simulink model "sm_DynamicCompression"  (R2019b)
settings: Solver=FixedStepDiscrete  StartTime=0.0  StopTime=stop_time  RelTol=1e-3
InitFcn:
  | sm_callback_init
StopFcn:
  | sm_callback_stop
values from neighbouring files (symbols this model uses):
  a = 100*(r^2)    [InitializeCompressionSettings.m]    (also in sm_check_control_signals.m = registers(i).(supplied_fields{j}); sm_check_control_signals_LOCAL_1434.m = registers(i).(supplied_fields{j}))
  B_k_0_init = zeros(1,FIR_0_Uprate)    [sm_callback_init.m]
  B_k_1_init = zeros(1,FIR_0_Uprate)    [sm_callback_init.m]
  B_k_2_init = zeros(1,FIR_0_Uprate)    [sm_callback_init.m]
  B_k_3_init = zeros(1,FIR_0_Uprate)    [sm_callback_init.m]
  B_k_4_init = zeros(1,FIR_0_Uprate)    [sm_callback_init.m]
  B_k_5_init = zeros(1,FIR_0_Uprate)    [sm_callback_init.m]
  calib_bpfs = bpfs    [sm_compression_init.m]
  delayFix = maxDelay-delays    [Initialize_Delay_Values.m]
  F_bits = 28    [TestingLibraryScripts.m]    (also in sm_compression_init.m)
  FIR_0_Size = (ceil(log2(length(calib_bpfs(2:calib_bpfs(1,1)+1 ,1)'))))    [sm_callback_init.m]
  FIR_0_Uprate = 2^FIR_0_Size    [sm_callback_init.m]
  M_bits = 1    [TestingLibraryScripts.m]    (also in sm_compression_init.m = 5)
  M_Bits = M_bits    (= 5)    [sm_compression_init.m]
  mp = sm_init_avalon_signals(mp)    [sm_callback_init.m]
  r_att = nthroot(0.1, s_att)    [sm_compression_init.m]
  r_rel = nthroot(0.1, s_rel)    [sm_compression_init.m]
  recombGain = ones(1,NChans)    [sm_compression_init.m]
  TABLE_SEL_BYPASS_ENABLE = 0    [sm_callback_init.m]
  Ts = mp.Ts    [sm_compression_init.m]
  Ts_system = mp.Ts_system    [sm_compression_init.m]
  W_bits = 32    [TestingLibraryScripts.m]    (also in sm_compression_init.m)
  X_high = 1    [sm_compression_init.m]
undefined symbols (not defined in the file or in its folder): b, c, Gain_Table, ig_eq
libraries: hdlsllib x272, simulink x127, dsphdlfiltering x2
(part 2 of 8)

== system sm_DynamicCompression/dataplane/Avalon Data Processing/Left Channel Processing/recalculate/Nchan_FbankAGC_AID/Static_pFIR2 ==
  note: consider desired output rate
  note: B_ks will be programmable eventually.
      | For the Conference, they will be preset.
  Data_In : Inport
  Valid_in : Inport  Port=2
  "Addr_Gen " : Subsystem
  Alignment_Delay : UnitDelay  SampleTime=-1  HasFrameUpgradeWarning=on
  Always_read_B2 : Constant  Value=0  OutDataTypeStr=boolean  SampleTime=Ts/FIR_0_Uprate
  B_k_Memory_Block : Subsystem  AncestorBlock=DualPortRam_UNLOCKED/Dual Rate Dual Port RAM1  mask(Dual-rate dual-port RAM){ram_size=FIR_0_Size}
      mask prompts: ram_size "Address port width (2 to 28 bits)"
      mask help: This block simulates a dual-clock dual-port RAM with two data output ports.
      mask init:
      | hdlblkmask_drdpram();
      mask Help: helpview([docroot '/simulink/helptargets.map'],'HDL_dual_rate_dual_port_ram');
  Input_Data_Circular_Buffer : hdlsllib/HDL RAMs/Simple Dual Port RAM  ram_size=FIR_0_Size
      settings: SourceProductName=Simulink  SourceProductBaseCode=SL
  Input_Data_Circular_Buffer_old : Subsystem  Commented=on  AncestorBlock=DualPortRam_UNLOCKED/Dual Rate Dual Port RAM1  mask(Dual-rate dual-port RAM){ram_size=FIR_0_Size}
      mask prompts: ram_size "Address port width (2 to 28 bits)"
      mask help: This block simulates a dual-clock dual-port RAM with two data output ports.
      mask init:
      | hdlblkmask_drdpram();
      mask Help: helpview([docroot '/simulink/helptargets.map'],'HDL_dual_rate_dual_port_ram');
  Multiply_And_Sum : Subsystem
  Never_write_B2 : Constant  Value=0  OutDataTypeStr=fixdt(1,W_bits, F_bits)  SampleTime=Ts/FIR_0_Uprate
  Output_memory : UnitDelay  SampleTime=-1  HasFrameUpgradeWarning=on
  READ_ONLY_1 : Constant  Value=0  OutDataTypeStr=fixdt(1,W_bits, F_bits)  SampleTime=Ts/FIR_0_Uprate
  READ_ONLY_2 : Constant  Value=0  OutDataTypeStr=fixdt(0,FIR_0_Size, 0)  SampleTime=Ts/FIR_0_Uprate
  READ_ONLY_3 : Constant  Value=0  OutDataTypeStr=boolean  SampleTime=Ts/FIR_0_Uprate
  Rate Transition : RateTransition  Commented=on  OutPortSampleTime=Ts
  Reset_Switch : Switch  Criteria=u2 ~= 0
  Terminator7 : Terminator
  Data_out : Outport  VectorParamsAs1DForOutWhenUnconnected=off
  wires:
  READ_ONLY_2/1 -> B_k_Memory_Block/2(addr_A)
  Always_read_B2/1 -> B_k_Memory_Block/6(we_B)
  B_k_Memory_Block/1(dout_A) -> Terminator7/1
  "Addr_Gen "/3(End_of_sample_calc) -> Alignment_Delay/1
  B_k_Memory_Block/2(dout_B) -> Multiply_And_Sum/3(b_i)  "b_i"
  Reset_Switch/1 -> Output_memory/1
  Multiply_And_Sum/2(Output_Valid) -> Reset_Switch/2
  READ_ONLY_1/1 -> B_k_Memory_Block/1(din_A)
  Never_write_B2/1 -> B_k_Memory_Block/4(din_B)
  Input_Data_Circular_Buffer/1 -> Multiply_And_Sum/1(x[n-i])  "x[n-i]"
  "Addr_Gen "/2(Data_History_Rd_addr) -> Input_Data_Circular_Buffer/4
  Valid_in/1 -> Input_Data_Circular_Buffer/3
  Output_memory/1 -> Data_out/1, Reset_Switch/3
  READ_ONLY_3/1 -> B_k_Memory_Block/3(we_A)
  "Addr_Gen "/1(Input_Addr) -> Input_Data_Circular_Buffer/2
  Multiply_And_Sum/1(Filtered_Output) -> Reset_Switch/1
  "Addr_Gen "/4(b_k_addr) -> B_k_Memory_Block/5(addr_B)
  Data_In/1 -> Input_Data_Circular_Buffer/1  "x[n]"
  Alignment_Delay/1 -> Multiply_And_Sum/2(End_of_sample_calc)

== system sm_DynamicCompression/dataplane/Avalon Data Processing/Left Channel Processing/recalculate/Nchan_FbankAGC_AID/Static_pFIR3 ==
  note: B_ks will be programmable eventually.
      | For the Conference, they will be preset.
  note: consider desired output rate
  Data_In : Inport
  Valid_in : Inport  Port=2
  "Addr_Gen " : Subsystem
  Alignment_Delay : UnitDelay  SampleTime=-1  HasFrameUpgradeWarning=on
  Always_read_B2 : Constant  Value=0  OutDataTypeStr=boolean  SampleTime=Ts/FIR_0_Uprate
  B_k_Memory_Block : Subsystem  AncestorBlock=DualPortRam_UNLOCKED/Dual Rate Dual Port RAM1  mask(Dual-rate dual-port RAM){ram_size=FIR_0_Size}
      mask prompts: ram_size "Address port width (2 to 28 bits)"
      mask help: This block simulates a dual-clock dual-port RAM with two data output ports.
      mask init:
      | hdlblkmask_drdpram();
      mask Help: helpview([docroot '/simulink/helptargets.map'],'HDL_dual_rate_dual_port_ram');
  Input_Data_Circular_Buffer : hdlsllib/HDL RAMs/Simple Dual Port RAM  ram_size=FIR_0_Size
      settings: SourceProductName=Simulink  SourceProductBaseCode=SL
  Input_Data_Circular_Buffer_old : Subsystem  Commented=on  AncestorBlock=DualPortRam_UNLOCKED/Dual Rate Dual Port RAM1  mask(Dual-rate dual-port RAM){ram_size=FIR_0_Size}
      mask prompts: ram_size "Address port width (2 to 28 bits)"
      mask help: This block simulates a dual-clock dual-port RAM with two data output ports.
      mask init:
      | hdlblkmask_drdpram();
      mask Help: helpview([docroot '/simulink/helptargets.map'],'HDL_dual_rate_dual_port_ram');
  Multiply_And_Sum : Subsystem
  Never_write_B2 : Constant  Value=0  OutDataTypeStr=fixdt(1,W_bits, F_bits)  SampleTime=Ts/FIR_0_Uprate
  Output_memory : UnitDelay  SampleTime=-1  HasFrameUpgradeWarning=on
  READ_ONLY_1 : Constant  Value=0  OutDataTypeStr=fixdt(1,W_bits, F_bits)  SampleTime=Ts/FIR_0_Uprate
  READ_ONLY_2 : Constant  Value=0  OutDataTypeStr=fixdt(0,FIR_0_Size, 0)  SampleTime=Ts/FIR_0_Uprate
  READ_ONLY_3 : Constant  Value=0  OutDataTypeStr=boolean  SampleTime=Ts/FIR_0_Uprate
  Rate Transition : RateTransition  Commented=on  OutPortSampleTime=Ts
  Reset_Switch : Switch  Criteria=u2 ~= 0
  Terminator7 : Terminator
  Data_out : Outport  VectorParamsAs1DForOutWhenUnconnected=off
  wires:
  Alignment_Delay/1 -> Multiply_And_Sum/2(End_of_sample_calc)
  Data_In/1 -> Input_Data_Circular_Buffer/1  "x[n]"
  "Addr_Gen "/4(b_k_addr) -> B_k_Memory_Block/5(addr_B)
  Multiply_And_Sum/1(Filtered_Output) -> Reset_Switch/1
  "Addr_Gen "/1(Input_Addr) -> Input_Data_Circular_Buffer/2
  READ_ONLY_3/1 -> B_k_Memory_Block/3(we_A)
  Output_memory/1 -> Reset_Switch/3, Data_out/1
  Valid_in/1 -> Input_Data_Circular_Buffer/3
  "Addr_Gen "/2(Data_History_Rd_addr) -> Input_Data_Circular_Buffer/4
  Input_Data_Circular_Buffer/1 -> Multiply_And_Sum/1(x[n-i])  "x[n-i]"
  Never_write_B2/1 -> B_k_Memory_Block/4(din_B)
  READ_ONLY_1/1 -> B_k_Memory_Block/1(din_A)
  Multiply_And_Sum/2(Output_Valid) -> Reset_Switch/2
  Reset_Switch/1 -> Output_memory/1
  B_k_Memory_Block/2(dout_B) -> Multiply_And_Sum/3(b_i)  "b_i"
  "Addr_Gen "/3(End_of_sample_calc) -> Alignment_Delay/1
  B_k_Memory_Block/1(dout_A) -> Terminator7/1
  Always_read_B2/1 -> B_k_Memory_Block/6(we_B)
  READ_ONLY_2/1 -> B_k_Memory_Block/2(addr_A)

== system sm_DynamicCompression/dataplane/Avalon Data Processing/Left Channel Processing/recalculate/Nchan_FbankAGC_AID/Static_pFIR4 ==
  note: consider desired output rate
  note: B_ks will be programmable eventually.
      | For the Conference, they will be preset.
  Data_In : Inport
  Valid_in : Inport  Port=2
  "Addr_Gen " : Subsystem
  Alignment_Delay : UnitDelay  SampleTime=-1  HasFrameUpgradeWarning=on
  Always_read_B2 : Constant  Value=0  OutDataTypeStr=boolean  SampleTime=Ts/FIR_0_Uprate
  B_k_Memory_Block : Subsystem  AncestorBlock=DualPortRam_UNLOCKED/Dual Rate Dual Port RAM1  mask(Dual-rate dual-port RAM){ram_size=FIR_0_Size}
      mask prompts: ram_size "Address port width (2 to 28 bits)"
      mask help: This block simulates a dual-clock dual-port RAM with two data output ports.
      mask init:
      | hdlblkmask_drdpram();
      mask Help: helpview([docroot '/simulink/helptargets.map'],'HDL_dual_rate_dual_port_ram');
  Input_Data_Circular_Buffer : hdlsllib/HDL RAMs/Simple Dual Port RAM  ram_size=FIR_0_Size
      settings: SourceProductName=Simulink  SourceProductBaseCode=SL
  Input_Data_Circular_Buffer_old : Subsystem  Commented=on  AncestorBlock=DualPortRam_UNLOCKED/Dual Rate Dual Port RAM1  mask(Dual-rate dual-port RAM){ram_size=FIR_0_Size}
      mask prompts: ram_size "Address port width (2 to 28 bits)"
      mask help: This block simulates a dual-clock dual-port RAM with two data output ports.
      mask init:
      | hdlblkmask_drdpram();
      mask Help: helpview([docroot '/simulink/helptargets.map'],'HDL_dual_rate_dual_port_ram');
  Multiply_And_Sum : Subsystem
  Never_write_B2 : Constant  Value=0  OutDataTypeStr=fixdt(1,W_bits, F_bits)  SampleTime=Ts/FIR_0_Uprate
  Output_memory : UnitDelay  SampleTime=-1  HasFrameUpgradeWarning=on
  READ_ONLY_1 : Constant  Value=0  OutDataTypeStr=fixdt(1,W_bits, F_bits)  SampleTime=Ts/FIR_0_Uprate
  READ_ONLY_2 : Constant  Value=0  OutDataTypeStr=fixdt(0,FIR_0_Size, 0)  SampleTime=Ts/FIR_0_Uprate
  READ_ONLY_3 : Constant  Value=0  OutDataTypeStr=boolean  SampleTime=Ts/FIR_0_Uprate
  Rate Transition : RateTransition  Commented=on  OutPortSampleTime=Ts
  Reset_Switch : Switch  Criteria=u2 ~= 0
  Terminator7 : Terminator
  Data_out : Outport  VectorParamsAs1DForOutWhenUnconnected=off
  wires:
  READ_ONLY_2/1 -> B_k_Memory_Block/2(addr_A)
  Always_read_B2/1 -> B_k_Memory_Block/6(we_B)
  B_k_Memory_Block/1(dout_A) -> Terminator7/1
  "Addr_Gen "/3(End_of_sample_calc) -> Alignment_Delay/1
  B_k_Memory_Block/2(dout_B) -> Multiply_And_Sum/3(b_i)  "b_i"
  Reset_Switch/1 -> Output_memory/1
  Multiply_And_Sum/2(Output_Valid) -> Reset_Switch/2
  READ_ONLY_1/1 -> B_k_Memory_Block/1(din_A)
  Never_write_B2/1 -> B_k_Memory_Block/4(din_B)
  Input_Data_Circular_Buffer/1 -> Multiply_And_Sum/1(x[n-i])  "x[n-i]"
  "Addr_Gen "/2(Data_History_Rd_addr) -> Input_Data_Circular_Buffer/4
  Valid_in/1 -> Input_Data_Circular_Buffer/3
  Output_memory/1 -> Data_out/1, Reset_Switch/3
  READ_ONLY_3/1 -> B_k_Memory_Block/3(we_A)
  "Addr_Gen "/1(Input_Addr) -> Input_Data_Circular_Buffer/2
  Multiply_And_Sum/1(Filtered_Output) -> Reset_Switch/1
  "Addr_Gen "/4(b_k_addr) -> B_k_Memory_Block/5(addr_B)
  Data_In/1 -> Input_Data_Circular_Buffer/1  "x[n]"
  Alignment_Delay/1 -> Multiply_And_Sum/2(End_of_sample_calc)

== system sm_DynamicCompression/dataplane/Avalon Data Processing/Left Channel Processing/recalculate/Static_pFIR/Addr_Gen  ==
  note: Realign Delay here?
  Add : Sum  OutDataTypeStr=Inherit: Same as first input
  Compare To Zero : simulink/Logic and Bit Operations/Compare To Zero  relop===  OutDataTypeStr=boolean  ZeroCross=off
  Constant : Constant  OutDataTypeStr=fixdt(0, FIR_0_Size,0)  SampleTime=-1
  Counter 0 to |b_k|-1 : simulink/Sources/Counter Free-Running  NumBits=FIR_0_Size  tsamp=Ts/FIR_0_Uprate
  Input_Addr_Counter : simulink/Sources/Counter Free-Running  NumBits=FIR_0_Size  tsamp=Ts
  Rate Transition : RateTransition  OutPortSampleTime=Ts/FIR_0_Uprate
  Realignment_delay : Constant  Value=0  OutDataTypeStr=fixdt(0, FIR_0_Size,0)  SampleTime=-1
  Subtract : Sum  Inputs=+--  OutDataTypeStr=Inherit: Same as first input
  Input_Addr : Outport  VectorParamsAs1DForOutWhenUnconnected=off
  Data_History_Rd_addr : Outport  Port=2  VectorParamsAs1DForOutWhenUnconnected=off
  End_of_sample_calc : Outport  Port=3  VectorParamsAs1DForOutWhenUnconnected=off
  b_k_addr : Outport  Port=4  VectorParamsAs1DForOutWhenUnconnected=off
  wires:
  Counter 0 to |b_k|-1/1 -> Subtract/2, Compare To Zero/1, b_k_addr/1
  Subtract/1 -> Data_History_Rd_addr/1
  Input_Addr_Counter/1 -> Rate Transition/1
  Add/1 -> Input_Addr/1
  Constant/1 -> Add/2
  Realignment_delay/1 -> Subtract/3
  Compare To Zero/1 -> End_of_sample_calc/1
  Rate Transition/1 -> Subtract/1, Add/1

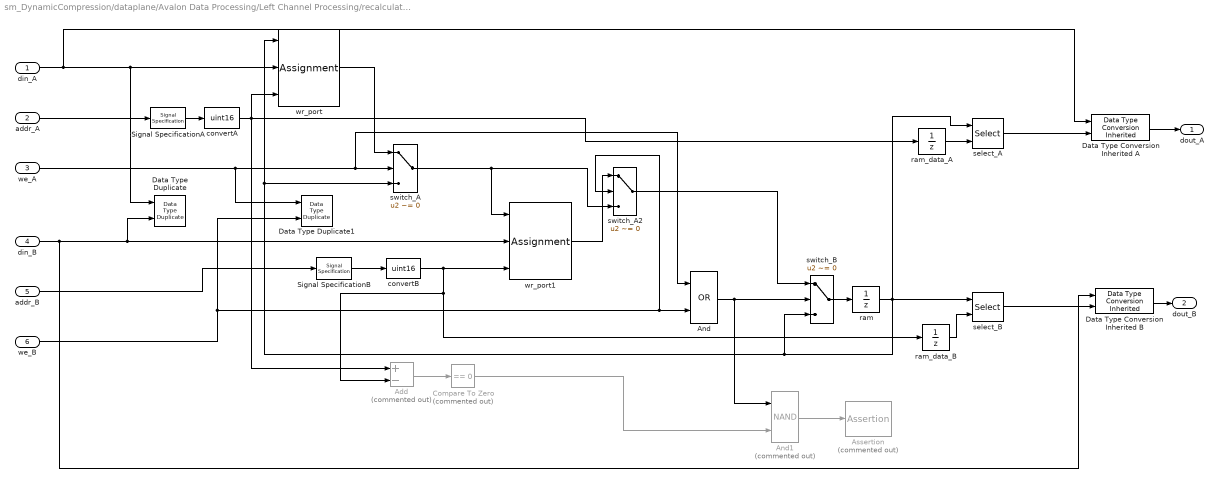
== system sm_DynamicCompression/dataplane/Avalon Data Processing/Left Channel Processing/recalculate/Static_pFIR/B_k_Memory_Block2 ==
  din_A : Inport
  addr_A : Inport  Port=2
  we_A : Inport  Port=3  OutDataTypeStr=boolean
  din_B : Inport  Port=4
  addr_B : Inport  Port=5
  we_B : Inport  Port=6  OutDataTypeStr=boolean
  Add : Sum  Commented=on  Inputs=+-
  And : Logic  Operator=OR  AllPortsSameDT=off  OutDataTypeStr=boolean
  And1 : Logic  Commented=on  Operator=NAND  AllPortsSameDT=off  OutDataTypeStr=boolean
  Assertion : Assertion  Commented=on  StopWhenAssertionFail=off
  Compare To Zero : simulink/Logic and Bit Operations/Compare To Zero  Commented=on  relop===  OutDataTypeStr=boolean
  Data Type Conversion Inherited A : simulink/Signal Attributes/Data Type Conversion Inherited  ConvertRealWorld=Real World Value  DoSatur=off
      settings: SourceProductName=Simulink  SourceProductBaseCode=SL
  Data Type Conversion Inherited B : simulink/Signal Attributes/Data Type Conversion Inherited  ConvertRealWorld=Real World Value  DoSatur=off
      settings: SourceProductName=Simulink  SourceProductBaseCode=SL
  Data Type Duplicate : DataTypeDuplicate
  Data Type Duplicate1 : DataTypeDuplicate
  Signal SpecificationA : SignalSpecification  OutDataTypeStr=fixdt(0,ram_size,0)  Dimensions=1
  Signal SpecificationB : SignalSpecification  OutDataTypeStr=fixdt(0,ram_size,0)  Dimensions=1
  convertA : DataTypeConversion  OutDataTypeStr=uint16
  convertB : DataTypeConversion  OutDataTypeStr=uint16
  ram : UnitDelay  InitialCondition=B_k_5_init  SampleTime=-1  HasFrameUpgradeWarning=on
  ram_data_A : UnitDelay  SampleTime=-1  HasFrameUpgradeWarning=on
  ram_data_B : UnitDelay  SampleTime=-1  HasFrameUpgradeWarning=on
  select_A : Selector  IndexMode=Zero-based  InputPortWidth=2^ram_size  IndexOptions=Index vector (port)  Indices=[1 3]  OutputSizes=1
  select_B : Selector  IndexMode=Zero-based  InputPortWidth=2^ram_size  IndexOptions=Index vector (port)  Indices=[1 3]  OutputSizes=1
  switch_A : Switch  Criteria=u2 ~= 0
  switch_A2 : Switch  Criteria=u2 ~= 0
  switch_B : Switch  Criteria=u2 ~= 0
  wr_port : Assignment  IndexMode=Zero-based  IndexOptions=Index vector (port)  Indices=1  OutputSizes=[1 1]
  wr_port1 : Assignment  IndexMode=Zero-based  IndexOptions=Index vector (port)  Indices=1  OutputSizes=[1 1]
  dout_A : Outport  VectorParamsAs1DForOutWhenUnconnected=off
  dout_B : Outport  Port=2  VectorParamsAs1DForOutWhenUnconnected=off
  wires:
  switch_A2/1 -> switch_B/1
  And1/1 -> Assertion/1
  Signal SpecificationA/1 -> convertA/1
  Signal SpecificationB/1 -> convertB/1
  switch_B/1 -> ram/1
  convertA/1 -> ram_data_A/1, wr_port/3, Add/1
  ram/1 -> select_B/1, switch_B/3, switch_A/3, wr_port/1, select_A/1
  wr_port/1 -> switch_A/1
  And/1 -> And1/1, switch_B/2
  wr_port1/1 -> switch_A2/1
  Add/1 -> Compare To Zero/1
  Compare To Zero/1 -> And1/2
  we_B/1 -> switch_A2/2, And/2, Data Type Duplicate1/2
  switch_A/1 -> wr_port1/1, switch_A2/3
  addr_B/1 -> Signal SpecificationB/1
  ram_data_B/1 -> select_B/2
  we_A/1 -> Data Type Duplicate1/1, And/1, switch_A/2
  ram_data_A/1 -> select_A/2
  din_A/1 -> Data Type Duplicate/1, wr_port/2, Data Type Conversion Inherited A/1
  convertB/1 -> ram_data_B/1, Add/2, wr_port1/3
  din_B/1 -> wr_port1/2, Data Type Duplicate/2, Data Type Conversion Inherited B/1
  addr_A/1 -> Signal SpecificationA/1
  select_B/1 -> Data Type Conversion Inherited B/2
  Data Type Conversion Inherited B/1 -> dout_B/1
  select_A/1 -> Data Type Conversion Inherited A/2
  Data Type Conversion Inherited A/1 -> dout_A/1

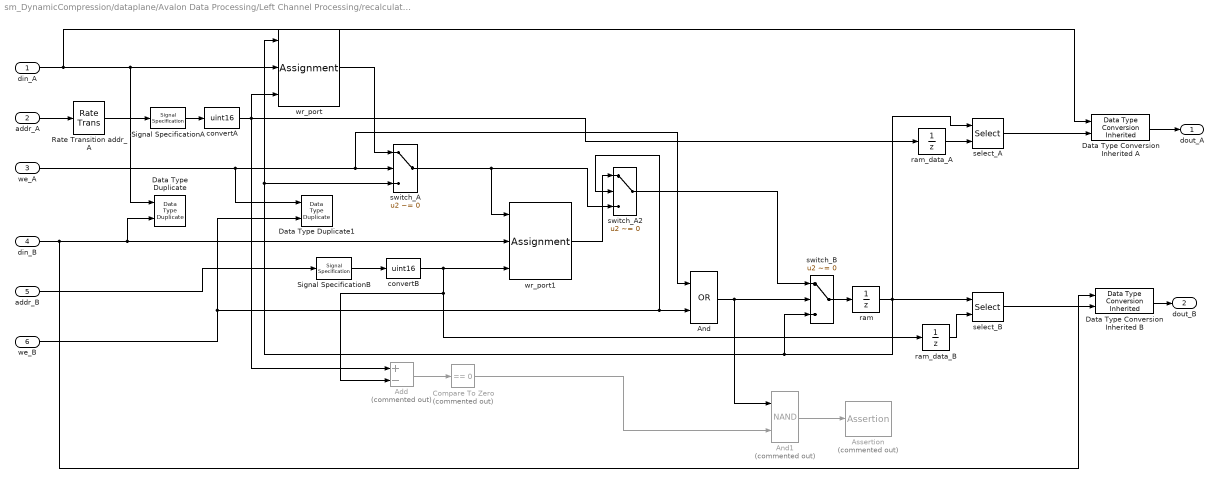
== system sm_DynamicCompression/dataplane/Avalon Data Processing/Left Channel Processing/recalculate/Static_pFIR/Input_Data_Circular_Buffer_old ==
  din_A : Inport
  addr_A : Inport  Port=2
  we_A : Inport  Port=3  OutDataTypeStr=boolean
  din_B : Inport  Port=4
  addr_B : Inport  Port=5
  we_B : Inport  Port=6  OutDataTypeStr=boolean
  Add : Sum  Commented=on  Inputs=+-
  And : Logic  Operator=OR  AllPortsSameDT=off  OutDataTypeStr=boolean
  And1 : Logic  Commented=on  Operator=NAND  AllPortsSameDT=off  OutDataTypeStr=boolean
  Assertion : Assertion  Commented=on  StopWhenAssertionFail=off
  Compare To Zero : simulink/Logic and Bit Operations/Compare To Zero  Commented=on  relop===  OutDataTypeStr=boolean
  Data Type Conversion Inherited A : simulink/Signal Attributes/Data Type Conversion Inherited  ConvertRealWorld=Real World Value  DoSatur=off
      settings: SourceProductName=Simulink  SourceProductBaseCode=SL
  Data Type Conversion Inherited B : simulink/Signal Attributes/Data Type Conversion Inherited  ConvertRealWorld=Real World Value  DoSatur=off
      settings: SourceProductName=Simulink  SourceProductBaseCode=SL
  Data Type Duplicate : DataTypeDuplicate
  Data Type Duplicate1 : DataTypeDuplicate
  Rate Transition addr_A : RateTransition
  Signal SpecificationA : SignalSpecification  OutDataTypeStr=fixdt(0,ram_size,0)  Dimensions=1
  Signal SpecificationB : SignalSpecification  OutDataTypeStr=fixdt(0,ram_size,0)  Dimensions=1
  convertA : DataTypeConversion  OutDataTypeStr=uint16
  convertB : DataTypeConversion  OutDataTypeStr=uint16
  ram : UnitDelay  SampleTime=-1  HasFrameUpgradeWarning=on
  ram_data_A : UnitDelay  SampleTime=-1  HasFrameUpgradeWarning=on
  ram_data_B : UnitDelay  SampleTime=-1  HasFrameUpgradeWarning=on
  select_A : Selector  IndexMode=Zero-based  InputPortWidth=2^ram_size  IndexOptions=Index vector (port)  Indices=[1 3]  OutputSizes=1
  select_B : Selector  IndexMode=Zero-based  InputPortWidth=2^ram_size  IndexOptions=Index vector (port)  Indices=[1 3]  OutputSizes=1
  switch_A : Switch  Criteria=u2 ~= 0
  switch_A2 : Switch  Criteria=u2 ~= 0
  switch_B : Switch  Criteria=u2 ~= 0
  wr_port : Assignment  IndexMode=Zero-based  IndexOptions=Index vector (port)  Indices=1  OutputSizes=[1 1]
  wr_port1 : Assignment  IndexMode=Zero-based  IndexOptions=Index vector (port)  Indices=1  OutputSizes=[1 1]
  dout_A : Outport  VectorParamsAs1DForOutWhenUnconnected=off
  dout_B : Outport  Port=2  VectorParamsAs1DForOutWhenUnconnected=off
  wires:
  Data Type Conversion Inherited A/1 -> dout_A/1
  select_A/1 -> Data Type Conversion Inherited A/2
  Data Type Conversion Inherited B/1 -> dout_B/1
  select_B/1 -> Data Type Conversion Inherited B/2
  Rate Transition addr_A/1 -> Signal SpecificationA/1
  addr_A/1 -> Rate Transition addr_A/1
  din_B/1 -> Data Type Duplicate/2, wr_port1/2, Data Type Conversion Inherited B/1
  convertB/1 -> wr_port1/3, Add/2, ram_data_B/1
  din_A/1 -> wr_port/2, Data Type Duplicate/1, Data Type Conversion Inherited A/1
  ram_data_A/1 -> select_A/2
  we_A/1 -> switch_A/2, And/1, Data Type Duplicate1/1
  ram_data_B/1 -> select_B/2
  addr_B/1 -> Signal SpecificationB/1
  switch_A/1 -> switch_A2/3, wr_port1/1
  we_B/1 -> Data Type Duplicate1/2, And/2, switch_A2/2
  Compare To Zero/1 -> And1/2
  Add/1 -> Compare To Zero/1
  wr_port1/1 -> switch_A2/1
  And/1 -> switch_B/2, And1/1
  wr_port/1 -> switch_A/1
  ram/1 -> select_A/1, wr_port/1, switch_A/3, switch_B/3, select_B/1
  convertA/1 -> Add/1, wr_port/3, ram_data_A/1
  switch_B/1 -> ram/1
  Signal SpecificationB/1 -> convertB/1
  Signal SpecificationA/1 -> convertA/1
  And1/1 -> Assertion/1
  switch_A2/1 -> switch_B/1

== system sm_DynamicCompression/dataplane/Avalon Data Processing/Left Channel Processing/recalculate/Static_pFIR/Multiply_And_Sum ==
  note: Try to use this at some point?
  note: End_of_sample_calc triggers this subsystem to give the FIR output for this sample.
      | Also, it resets the sum memory back to 0.
  x[n-i] : Inport
  End_of_sample_calc : Inport  Port=2
  b_i : Inport  Port=3
  Bitwise Operator : simulink/Logic and Bit Operations/Bitwise Operator  logicop=NOT  UseBitMask=off  BitMask=bin2dec('11011001')  BitMaskRealWorld=Stored Integer
  Constant : Constant  Value=0  OutDataTypeStr=fixdt(1, W_bits, F_bits)  SampleTime=Ts/FIR_0_Uprate
  Multiply-Add : hdlsllib/HDL Operations/Multiply-Add  Function=c+(a.*b)  datatype=Inherit: Same as first input  DoSatur=off  FMA=off
      settings: SourceProductName=Simulink  SourceProductBaseCode=SL
  Reset_Switch : Switch  Criteria=u2 ~= 0  ZeroCross=off
  Sum_memory : UnitDelay  SampleTime=-1  HasFrameUpgradeWarning=on
  convertB : DataTypeConversion  OutDataTypeStr=fixdt(1, W_bits, F_bits)
  Filtered_Output : Outport  VectorParamsAs1DForOutWhenUnconnected=off
  Output_Valid : Outport  Port=2  VectorParamsAs1DForOutWhenUnconnected=off
  wires:
  x[n-i]/1 -> Multiply-Add/1
  End_of_sample_calc/1 -> Output_Valid/1, Bitwise Operator/1
  b_i/1 -> Multiply-Add/2
  Sum_memory/1 -> Multiply-Add/3, Filtered_Output/1
  Multiply-Add/1 -> convertB/1
  Reset_Switch/1 -> Sum_memory/1
  Constant/1 -> Reset_Switch/3
  Bitwise Operator/1 -> Reset_Switch/2
  convertB/1 -> Reset_Switch/1

== system sm_DynamicCompression/dataplane/Avalon Data Processing/Left Channel Processing/recalculate/Nchan_FbankAGC_AID/Compression_1/Compression_Envelope ==
  note: Curr > Desired:
      | Attack
  note: Curr < Desired:
      | Release
  Desired_Gain : Inport
  Curr_Gain : Inport  Port=2
  Attack_Envelope : Subsystem  TreatAsAtomicUnit=on
  Compare To Zero : simulink/Logic and Bit Operations/Compare To Zero  relop=>=  OutDataTypeStr=boolean
  Logical Operator : Logic  Operator=NOT  AllPortsSameDT=off  OutDataTypeStr=boolean
  Release_Envelope : Subsystem  TreatAsAtomicUnit=on
  Subtract : Sum  Inputs=-+  AccumDataTypeStr=fixdt(1,W_bits,F_bits)  OutDataTypeStr=Inherit: Same as accumulator
  Switch : Switch
  Gain_Out : Outport  SampleTime=Ts  VectorParamsAs1DForOutWhenUnconnected=off
  wires:
  Desired_Gain/1 -> Attack_Envelope/2(Desired), Release_Envelope/2(Desired), Subtract/1
  Curr_Gain/1 -> Attack_Envelope/1(Curr), Subtract/2, Release_Envelope/1(Curr)
  Subtract/1 -> Switch/2, Compare To Zero/1
  Compare To Zero/1 -> Attack_Envelope/Enable, Logical Operator/1
  Logical Operator/1 -> Release_Envelope/Enable
  Switch/1 -> Gain_Out/1
  Attack_Envelope/1(Gain_out) -> Switch/1
  Release_Envelope/1(Gain_out) -> Switch/3

== system sm_DynamicCompression/dataplane/Avalon Data Processing/Left Channel Processing/recalculate/Nchan_FbankAGC_AID/Compression_1/Compression_Gain_Calc ==
  note: Data_In assumed before applied prescription FIR
  note: Compression: Assume the input is a single band coming from the system.
      |
      | Goals:
      | 	- Take in a single point
      | 	- compare the volume to a known hard cap for the data
      | 	- attenuate the signal if it's above a certain threshold
      | 		- the distance above the threshold should be cut in dB by a ratio R
      | 	- return the output point at the same sample rate received
  Table_Fill : Inport
  Write_Addr : Inport  Port=2
  Table_Fill_Valid : Inport  Port=3
  Data_In : Inport  Port=4
  Abs : Abs
  Constant : Constant  OutDataTypeStr=fixdt(0,9,0)  SampleTime=-1
  High_Gain_Table : Subsystem  AncestorBlock=DualPortRam_UNLOCKED/Dual Port RAM UNLOCKED  mask(Dual-port RAM){ram_size=4+M_bits}
      mask prompts: ram_size "Address port width (2 to 29 bits)"
      mask help: This block simulates a dual-port RAM with two data output ports.
      mask init:
      | hdlblkmask_dpram;
      mask Help: helpview([docroot '/simulink/helptargets.map'],'HDL_dual_port_RAM');
  Linear_Approximation : Subsystem
  LogAddressing : Subsystem
  Low_Gain_Table : Subsystem  AncestorBlock=DualPortRam_UNLOCKED/Dual Port RAM UNLOCKED  mask(Dual-port RAM){ram_size=4+M_bits}
      mask prompts: ram_size "Address port width (2 to 29 bits)"
      mask help: This block simulates a dual-port RAM with two data output ports.
      mask init:
      | hdlblkmask_dpram;
      mask Help: helpview([docroot '/simulink/helptargets.map'],'HDL_dual_port_RAM');
  Subtract : Sum  OutDataTypeStr=Inherit: Same as first input
  Terminator : Terminator
  Terminator1 : Terminator
  Unit Delay1 : UnitDelay  InitialCondition=1  SampleTime=-1  HasFrameUpgradeWarning=on
  Unit Delay2 : UnitDelay  InitialCondition=1  SampleTime=-1  HasFrameUpgradeWarning=on
  Unit Delay3 : UnitDelay  InitialCondition=1  SampleTime=-1  HasFrameUpgradeWarning=on
  Gain_C_out : Outport  VectorParamsAs1DForOutWhenUnconnected=off
  wires:
  Table_Fill/1 -> Low_Gain_Table/1(wr_din), High_Gain_Table/1(wr_din)
  Table_Fill_Valid/1 -> Low_Gain_Table/3(wr_en), High_Gain_Table/3(wr_en)
  Write_Addr/1 -> Low_Gain_Table/2(wr_addr), High_Gain_Table/2(wr_addr)
  LogAddressing/1(addr_r) -> Low_Gain_Table/4(rd_addr), Unit Delay3/1, Subtract/1  "addr_low"
  Abs/1 -> Unit Delay2/1, LogAddressing/1(x_in)  "|X_in|"
  Data_In/1 -> Abs/1
  Constant/1 -> Subtract/2
  Subtract/1 -> High_Gain_Table/4(rd_addr)  "addr_high"
  Low_Gain_Table/1(wr_dout) -> Terminator/1
  High_Gain_Table/1(wr_dout) -> Terminator1/1
  High_Gain_Table/2(rd_dout) -> Linear_Approximation/1(G_high)  "G_high"
  Low_Gain_Table/2(rd_dout) -> Linear_Approximation/2(G_low)  "G_low"
  Linear_Approximation/1(G_Desired) -> Gain_C_out/1
  Unit Delay2/1 -> Unit Delay1/1
  Unit Delay1/1 -> Linear_Approximation/4(|X_in|)
  Unit Delay3/1 -> Linear_Approximation/3(addr_low)

== system sm_DynamicCompression/dataplane/Avalon Data Processing/Left Channel Processing/recalculate/Nchan_FbankAGC_AID/Compression_2/Compression_Envelope ==
  note: Curr > Desired:
      | Attack
  note: Curr < Desired:
      | Release
  Desired_Gain : Inport
  Curr_Gain : Inport  Port=2
  Attack_Envelope : Subsystem  TreatAsAtomicUnit=on
  Compare To Zero : simulink/Logic and Bit Operations/Compare To Zero  relop=>=  OutDataTypeStr=boolean
  Logical Operator : Logic  Operator=NOT  AllPortsSameDT=off  OutDataTypeStr=boolean
  Release_Envelope : Subsystem  TreatAsAtomicUnit=on
  Subtract : Sum  Inputs=-+  AccumDataTypeStr=fixdt(1,W_bits,F_bits)  OutDataTypeStr=Inherit: Same as accumulator
  Switch : Switch
  Gain_Out : Outport  SampleTime=Ts  VectorParamsAs1DForOutWhenUnconnected=off
  wires:
  Desired_Gain/1 -> Attack_Envelope/2(Desired), Release_Envelope/2(Desired), Subtract/1
  Curr_Gain/1 -> Attack_Envelope/1(Curr), Subtract/2, Release_Envelope/1(Curr)
  Subtract/1 -> Switch/2, Compare To Zero/1
  Compare To Zero/1 -> Attack_Envelope/Enable, Logical Operator/1
  Logical Operator/1 -> Release_Envelope/Enable
  Switch/1 -> Gain_Out/1
  Attack_Envelope/1(Gain_out) -> Switch/1
  Release_Envelope/1(Gain_out) -> Switch/3

== system sm_DynamicCompression/dataplane/Avalon Data Processing/Left Channel Processing/recalculate/Nchan_FbankAGC_AID/Compression_2/Compression_Gain_Calc ==
  note: Data_In assumed before applied prescription FIR
  note: Compression: Assume the input is a single band coming from the system.
      |
      | Goals:
      | 	- Take in a single point
      | 	- compare the volume to a known hard cap for the data
      | 	- attenuate the signal if it's above a certain threshold
      | 		- the distance above the threshold should be cut in dB by a ratio R
      | 	- return the output point at the same sample rate received
  Table_Fill : Inport
  Write_Addr : Inport  Port=2
  Table_Fill_Valid : Inport  Port=3
  Data_In : Inport  Port=4
  Abs : Abs
  Constant : Constant  OutDataTypeStr=fixdt(0,9,0)  SampleTime=-1
  High_Gain_Table : Subsystem  AncestorBlock=DualPortRam_UNLOCKED/Dual Port RAM UNLOCKED  mask(Dual-port RAM){ram_size=4+M_bits}
      mask prompts: ram_size "Address port width (2 to 29 bits)"
      mask help: This block simulates a dual-port RAM with two data output ports.
      mask init:
      | hdlblkmask_dpram;
      mask Help: helpview([docroot '/simulink/helptargets.map'],'HDL_dual_port_RAM');
  Linear_Approximation : Subsystem
  LogAddressing : Subsystem
  Low_Gain_Table : Subsystem  AncestorBlock=DualPortRam_UNLOCKED/Dual Port RAM UNLOCKED  mask(Dual-port RAM){ram_size=4+M_bits}
      mask prompts: ram_size "Address port width (2 to 29 bits)"
      mask help: This block simulates a dual-port RAM with two data output ports.
      mask init:
      | hdlblkmask_dpram;
      mask Help: helpview([docroot '/simulink/helptargets.map'],'HDL_dual_port_RAM');
  Subtract : Sum  OutDataTypeStr=Inherit: Same as first input
  Terminator : Terminator
  Terminator1 : Terminator
  Unit Delay1 : UnitDelay  InitialCondition=1  SampleTime=-1  HasFrameUpgradeWarning=on
  Unit Delay2 : UnitDelay  InitialCondition=1  SampleTime=-1  HasFrameUpgradeWarning=on
  Unit Delay3 : UnitDelay  InitialCondition=1  SampleTime=-1  HasFrameUpgradeWarning=on
  Gain_C_out : Outport  VectorParamsAs1DForOutWhenUnconnected=off
  wires:
  Table_Fill/1 -> Low_Gain_Table/1(wr_din), High_Gain_Table/1(wr_din)
  Table_Fill_Valid/1 -> Low_Gain_Table/3(wr_en), High_Gain_Table/3(wr_en)
  Write_Addr/1 -> Low_Gain_Table/2(wr_addr), High_Gain_Table/2(wr_addr)
  LogAddressing/1(addr_r) -> Low_Gain_Table/4(rd_addr), Unit Delay3/1, Subtract/1  "addr_low"
  Abs/1 -> LogAddressing/1(x_in), Unit Delay2/1  "|X_in|"
  Data_In/1 -> Abs/1
  Constant/1 -> Subtract/2
  Subtract/1 -> High_Gain_Table/4(rd_addr)  "addr_high"
  Low_Gain_Table/1(wr_dout) -> Terminator/1
  High_Gain_Table/1(wr_dout) -> Terminator1/1
  High_Gain_Table/2(rd_dout) -> Linear_Approximation/1(G_high)  "G_high"
  Low_Gain_Table/2(rd_dout) -> Linear_Approximation/2(G_low)  "G_low"
  Linear_Approximation/1(G_Desired) -> Gain_C_out/1
  Unit Delay2/1 -> Unit Delay1/1
  Unit Delay1/1 -> Linear_Approximation/4(|X_in|)
  Unit Delay3/1 -> Linear_Approximation/3(addr_low)

== system sm_DynamicCompression/dataplane/Avalon Data Processing/Left Channel Processing/recalculate/Nchan_FbankAGC_AID/Compression_3/Compression_Envelope ==
  note: Curr > Desired:
      | Attack
  note: Curr < Desired:
      | Release
  Desired_Gain : Inport
  Curr_Gain : Inport  Port=2
  Attack_Envelope : Subsystem  TreatAsAtomicUnit=on
  Compare To Zero : simulink/Logic and Bit Operations/Compare To Zero  relop=>=  OutDataTypeStr=boolean
  Logical Operator : Logic  Operator=NOT  AllPortsSameDT=off  OutDataTypeStr=boolean
  Release_Envelope : Subsystem  TreatAsAtomicUnit=on
  Subtract : Sum  Inputs=-+  AccumDataTypeStr=fixdt(1,W_bits,F_bits)  OutDataTypeStr=Inherit: Same as accumulator
  Switch : Switch
  Gain_Out : Outport  SampleTime=Ts  VectorParamsAs1DForOutWhenUnconnected=off
  wires:
  Desired_Gain/1 -> Attack_Envelope/2(Desired), Release_Envelope/2(Desired), Subtract/1
  Curr_Gain/1 -> Attack_Envelope/1(Curr), Subtract/2, Release_Envelope/1(Curr)
  Subtract/1 -> Switch/2, Compare To Zero/1
  Compare To Zero/1 -> Attack_Envelope/Enable, Logical Operator/1
  Logical Operator/1 -> Release_Envelope/Enable
  Switch/1 -> Gain_Out/1
  Attack_Envelope/1(Gain_out) -> Switch/1
  Release_Envelope/1(Gain_out) -> Switch/3

== system sm_DynamicCompression/dataplane/Avalon Data Processing/Left Channel Processing/recalculate/Nchan_FbankAGC_AID/Compression_3/Compression_Gain_Calc ==
  note: Data_In assumed before applied prescription FIR
  note: Compression: Assume the input is a single band coming from the system.
      |
      | Goals:
      | 	- Take in a single point
      | 	- compare the volume to a known hard cap for the data
      | 	- attenuate the signal if it's above a certain threshold
      | 		- the distance above the threshold should be cut in dB by a ratio R
      | 	- return the output point at the same sample rate received
  Table_Fill : Inport
  Write_Addr : Inport  Port=2
  Table_Fill_Valid : Inport  Port=3
  Data_In : Inport  Port=4
  Abs : Abs
  Constant : Constant  OutDataTypeStr=fixdt(0,9,0)  SampleTime=-1
  High_Gain_Table : Subsystem  AncestorBlock=DualPortRam_UNLOCKED/Dual Port RAM UNLOCKED  mask(Dual-port RAM){ram_size=4+M_bits}
      mask prompts: ram_size "Address port width (2 to 29 bits)"
      mask help: This block simulates a dual-port RAM with two data output ports.
      mask init:
      | hdlblkmask_dpram;
      mask Help: helpview([docroot '/simulink/helptargets.map'],'HDL_dual_port_RAM');
  Linear_Approximation : Subsystem
  LogAddressing : Subsystem
  Low_Gain_Table : Subsystem  AncestorBlock=DualPortRam_UNLOCKED/Dual Port RAM UNLOCKED  mask(Dual-port RAM){ram_size=4+M_bits}
      mask prompts: ram_size "Address port width (2 to 29 bits)"
      mask help: This block simulates a dual-port RAM with two data output ports.
      mask init:
      | hdlblkmask_dpram;
      mask Help: helpview([docroot '/simulink/helptargets.map'],'HDL_dual_port_RAM');
  Subtract : Sum  OutDataTypeStr=Inherit: Same as first input
  Terminator : Terminator
  Terminator1 : Terminator
  Unit Delay1 : UnitDelay  InitialCondition=1  SampleTime=-1  HasFrameUpgradeWarning=on
  Unit Delay2 : UnitDelay  InitialCondition=1  SampleTime=-1  HasFrameUpgradeWarning=on
  Unit Delay3 : UnitDelay  InitialCondition=1  SampleTime=-1  HasFrameUpgradeWarning=on
  Gain_C_out : Outport  VectorParamsAs1DForOutWhenUnconnected=off
  wires:
  Table_Fill/1 -> Low_Gain_Table/1(wr_din), High_Gain_Table/1(wr_din)
  Table_Fill_Valid/1 -> Low_Gain_Table/3(wr_en), High_Gain_Table/3(wr_en)
  Write_Addr/1 -> Low_Gain_Table/2(wr_addr), High_Gain_Table/2(wr_addr)
  LogAddressing/1(addr_r) -> Low_Gain_Table/4(rd_addr), Unit Delay3/1, Subtract/1  "addr_low"
  Abs/1 -> LogAddressing/1(x_in), Unit Delay2/1  "|X_in|"
  Data_In/1 -> Abs/1
  Constant/1 -> Subtract/2
  Subtract/1 -> High_Gain_Table/4(rd_addr)  "addr_high"
  Low_Gain_Table/1(wr_dout) -> Terminator/1
  High_Gain_Table/1(wr_dout) -> Terminator1/1
  High_Gain_Table/2(rd_dout) -> Linear_Approximation/1(G_high)  "G_high"
  Low_Gain_Table/2(rd_dout) -> Linear_Approximation/2(G_low)  "G_low"
  Linear_Approximation/1(G_Desired) -> Gain_C_out/1
  Unit Delay2/1 -> Unit Delay1/1
  Unit Delay1/1 -> Linear_Approximation/4(|X_in|)
  Unit Delay3/1 -> Linear_Approximation/3(addr_low)

== system sm_DynamicCompression/dataplane/Avalon Data Processing/Left Channel Processing/recalculate/Nchan_FbankAGC_AID/Compression_4/Compression_Envelope ==
  note: Curr > Desired:
      | Attack
  note: Curr < Desired:
      | Release
  Desired_Gain : Inport
  Curr_Gain : Inport  Port=2
  Attack_Envelope : Subsystem  TreatAsAtomicUnit=on
  Compare To Zero : simulink/Logic and Bit Operations/Compare To Zero  relop=>=  OutDataTypeStr=boolean
  Logical Operator : Logic  Operator=NOT  AllPortsSameDT=off  OutDataTypeStr=boolean
  Release_Envelope : Subsystem  TreatAsAtomicUnit=on
  Subtract : Sum  Inputs=-+  AccumDataTypeStr=fixdt(1,W_bits,F_bits)  OutDataTypeStr=Inherit: Same as accumulator
  Switch : Switch
  Gain_Out : Outport  SampleTime=Ts  VectorParamsAs1DForOutWhenUnconnected=off
  wires:
  Desired_Gain/1 -> Attack_Envelope/2(Desired), Release_Envelope/2(Desired), Subtract/1
  Curr_Gain/1 -> Attack_Envelope/1(Curr), Subtract/2, Release_Envelope/1(Curr)
  Subtract/1 -> Switch/2, Compare To Zero/1
  Compare To Zero/1 -> Attack_Envelope/Enable, Logical Operator/1
  Logical Operator/1 -> Release_Envelope/Enable
  Switch/1 -> Gain_Out/1
  Attack_Envelope/1(Gain_out) -> Switch/1
  Release_Envelope/1(Gain_out) -> Switch/3

== system sm_DynamicCompression/dataplane/Avalon Data Processing/Left Channel Processing/recalculate/Nchan_FbankAGC_AID/Compression_4/Compression_Gain_Calc ==
  note: Data_In assumed before applied prescription FIR
  note: Compression: Assume the input is a single band coming from the system.
      |
      | Goals:
      | 	- Take in a single point
      | 	- compare the volume to a known hard cap for the data
      | 	- attenuate the signal if it's above a certain threshold
      | 		- the distance above the threshold should be cut in dB by a ratio R
      | 	- return the output point at the same sample rate received
  Table_Fill : Inport
  Write_Addr : Inport  Port=2
  Table_Fill_Valid : Inport  Port=3
  Data_In : Inport  Port=4
  Abs : Abs
  Constant : Constant  OutDataTypeStr=fixdt(0,9,0)  SampleTime=-1
  High_Gain_Table : Subsystem  AncestorBlock=DualPortRam_UNLOCKED/Dual Port RAM UNLOCKED  mask(Dual-port RAM){ram_size=4+M_bits}
      mask prompts: ram_size "Address port width (2 to 29 bits)"
      mask help: This block simulates a dual-port RAM with two data output ports.
      mask init:
      | hdlblkmask_dpram;
      mask Help: helpview([docroot '/simulink/helptargets.map'],'HDL_dual_port_RAM');
  Linear_Approximation : Subsystem
  LogAddressing : Subsystem
  Low_Gain_Table : Subsystem  AncestorBlock=DualPortRam_UNLOCKED/Dual Port RAM UNLOCKED  mask(Dual-port RAM){ram_size=4+M_bits}
      mask prompts: ram_size "Address port width (2 to 29 bits)"
      mask help: This block simulates a dual-port RAM with two data output ports.
      mask init:
      | hdlblkmask_dpram;
      mask Help: helpview([docroot '/simulink/helptargets.map'],'HDL_dual_port_RAM');
  Subtract : Sum  OutDataTypeStr=Inherit: Same as first input
  Terminator : Terminator
  Terminator1 : Terminator
  Unit Delay1 : UnitDelay  InitialCondition=1  SampleTime=-1  HasFrameUpgradeWarning=on
  Unit Delay2 : UnitDelay  InitialCondition=1  SampleTime=-1  HasFrameUpgradeWarning=on
  Unit Delay3 : UnitDelay  InitialCondition=1  SampleTime=-1  HasFrameUpgradeWarning=on
  Gain_C_out : Outport  VectorParamsAs1DForOutWhenUnconnected=off
  wires:
  Table_Fill/1 -> Low_Gain_Table/1(wr_din), High_Gain_Table/1(wr_din)
  Table_Fill_Valid/1 -> Low_Gain_Table/3(wr_en), High_Gain_Table/3(wr_en)
  Write_Addr/1 -> Low_Gain_Table/2(wr_addr), High_Gain_Table/2(wr_addr)
  LogAddressing/1(addr_r) -> Low_Gain_Table/4(rd_addr), Unit Delay3/1, Subtract/1  "addr_low"
  Abs/1 -> LogAddressing/1(x_in), Unit Delay2/1  "|X_in|"
  Data_In/1 -> Abs/1
  Constant/1 -> Subtract/2
  Subtract/1 -> High_Gain_Table/4(rd_addr)  "addr_high"
  Low_Gain_Table/1(wr_dout) -> Terminator/1
  High_Gain_Table/1(wr_dout) -> Terminator1/1
  High_Gain_Table/2(rd_dout) -> Linear_Approximation/1(G_high)  "G_high"
  Low_Gain_Table/2(rd_dout) -> Linear_Approximation/2(G_low)  "G_low"
  Linear_Approximation/1(G_Desired) -> Gain_C_out/1
  Unit Delay2/1 -> Unit Delay1/1
  Unit Delay1/1 -> Linear_Approximation/4(|X_in|)
  Unit Delay3/1 -> Linear_Approximation/3(addr_low)

== system sm_DynamicCompression/dataplane/Avalon Data Processing/Left Channel Processing/recalculate/Nchan_FbankAGC_AID/Compression_5/Compression_Envelope ==
  note: Curr > Desired:
      | Attack
  note: Curr < Desired:
      | Release
  Desired_Gain : Inport
  Curr_Gain : Inport  Port=2
  Attack_Envelope : Subsystem  TreatAsAtomicUnit=on
  Compare To Zero : simulink/Logic and Bit Operations/Compare To Zero  relop=>=  OutDataTypeStr=boolean
  Logical Operator : Logic  Operator=NOT  AllPortsSameDT=off  OutDataTypeStr=boolean
  Release_Envelope : Subsystem  TreatAsAtomicUnit=on
  Subtract : Sum  Inputs=-+  AccumDataTypeStr=fixdt(1,W_bits,F_bits)  OutDataTypeStr=Inherit: Same as accumulator
  Switch : Switch
  Gain_Out : Outport  SampleTime=Ts  VectorParamsAs1DForOutWhenUnconnected=off
  wires:
  Desired_Gain/1 -> Attack_Envelope/2(Desired), Release_Envelope/2(Desired), Subtract/1
  Curr_Gain/1 -> Attack_Envelope/1(Curr), Subtract/2, Release_Envelope/1(Curr)
  Subtract/1 -> Switch/2, Compare To Zero/1
  Compare To Zero/1 -> Attack_Envelope/Enable, Logical Operator/1
  Logical Operator/1 -> Release_Envelope/Enable
  Switch/1 -> Gain_Out/1
  Attack_Envelope/1(Gain_out) -> Switch/1
  Release_Envelope/1(Gain_out) -> Switch/3

== system sm_DynamicCompression/dataplane/Avalon Data Processing/Left Channel Processing/recalculate/Nchan_FbankAGC_AID/Compression_5/Compression_Gain_Calc ==
  note: Data_In assumed before applied prescription FIR
  note: Compression: Assume the input is a single band coming from the system.
      |
      | Goals:
      | 	- Take in a single point
      | 	- compare the volume to a known hard cap for the data
      | 	- attenuate the signal if it's above a certain threshold
      | 		- the distance above the threshold should be cut in dB by a ratio R
      | 	- return the output point at the same sample rate received
  Table_Fill : Inport
  Write_Addr : Inport  Port=2
  Table_Fill_Valid : Inport  Port=3
  Data_In : Inport  Port=4
  Abs : Abs
  Constant : Constant  OutDataTypeStr=fixdt(0,9,0)  SampleTime=-1
  High_Gain_Table : Subsystem  AncestorBlock=DualPortRam_UNLOCKED/Dual Port RAM UNLOCKED  mask(Dual-port RAM){ram_size=4+M_bits}
      mask prompts: ram_size "Address port width (2 to 29 bits)"
      mask help: This block simulates a dual-port RAM with two data output ports.
      mask init:
      | hdlblkmask_dpram;
      mask Help: helpview([docroot '/simulink/helptargets.map'],'HDL_dual_port_RAM');
  Linear_Approximation : Subsystem
  LogAddressing : Subsystem
  Low_Gain_Table : Subsystem  AncestorBlock=DualPortRam_UNLOCKED/Dual Port RAM UNLOCKED  mask(Dual-port RAM){ram_size=4+M_bits}
      mask prompts: ram_size "Address port width (2 to 29 bits)"
      mask help: This block simulates a dual-port RAM with two data output ports.
      mask init:
      | hdlblkmask_dpram;
      mask Help: helpview([docroot '/simulink/helptargets.map'],'HDL_dual_port_RAM');
  Subtract : Sum  OutDataTypeStr=Inherit: Same as first input
  Terminator : Terminator
  Terminator1 : Terminator
  Unit Delay1 : UnitDelay  InitialCondition=1  SampleTime=-1  HasFrameUpgradeWarning=on
  Unit Delay2 : UnitDelay  InitialCondition=1  SampleTime=-1  HasFrameUpgradeWarning=on
  Unit Delay3 : UnitDelay  InitialCondition=1  SampleTime=-1  HasFrameUpgradeWarning=on
  Gain_C_out : Outport  VectorParamsAs1DForOutWhenUnconnected=off
  wires:
  Table_Fill/1 -> Low_Gain_Table/1(wr_din), High_Gain_Table/1(wr_din)
  Table_Fill_Valid/1 -> Low_Gain_Table/3(wr_en), High_Gain_Table/3(wr_en)
  Write_Addr/1 -> Low_Gain_Table/2(wr_addr), High_Gain_Table/2(wr_addr)
  LogAddressing/1(addr_r) -> Low_Gain_Table/4(rd_addr), Unit Delay3/1, Subtract/1  "addr_low"
  Abs/1 -> LogAddressing/1(x_in), Unit Delay2/1  "|X_in|"
  Data_In/1 -> Abs/1
  Constant/1 -> Subtract/2
  Subtract/1 -> High_Gain_Table/4(rd_addr)  "addr_high"
  Low_Gain_Table/1(wr_dout) -> Terminator/1
  High_Gain_Table/1(wr_dout) -> Terminator1/1
  High_Gain_Table/2(rd_dout) -> Linear_Approximation/1(G_high)  "G_high"
  Low_Gain_Table/2(rd_dout) -> Linear_Approximation/2(G_low)  "G_low"
  Linear_Approximation/1(G_Desired) -> Gain_C_out/1
  Unit Delay2/1 -> Unit Delay1/1
  Unit Delay1/1 -> Linear_Approximation/4(|X_in|)
  Unit Delay3/1 -> Linear_Approximation/3(addr_low)

== system sm_DynamicCompression/dataplane/Avalon Data Processing/Left Channel Processing/recalculate/Nchan_FbankAGC_AID/Static_pFIR/Addr_Gen  ==
  note: Realign Delay here?
  Add : Sum  OutDataTypeStr=Inherit: Same as first input
  Compare To Zero : simulink/Logic and Bit Operations/Compare To Zero  relop===  OutDataTypeStr=boolean  ZeroCross=off
  Constant : Constant  OutDataTypeStr=fixdt(0, FIR_0_Size,0)  SampleTime=-1
  Counter 0 to |b_k|-1 : simulink/Sources/Counter Free-Running  NumBits=FIR_0_Size  tsamp=Ts/FIR_0_Uprate
  Input_Addr_Counter : simulink/Sources/Counter Free-Running  NumBits=FIR_0_Size  tsamp=Ts
  Rate Transition : RateTransition  OutPortSampleTime=Ts/FIR_0_Uprate
  Realignment_delay : Constant  Value=delayFix(1)  OutDataTypeStr=fixdt(0, FIR_0_Size,0)  SampleTime=-1
  Subtract : Sum  Inputs=+--  OutDataTypeStr=Inherit: Same as first input
  Input_Addr : Outport  VectorParamsAs1DForOutWhenUnconnected=off
  Data_History_Rd_addr : Outport  Port=2  VectorParamsAs1DForOutWhenUnconnected=off
  End_of_sample_calc : Outport  Port=3  VectorParamsAs1DForOutWhenUnconnected=off
  b_k_addr : Outport  Port=4  VectorParamsAs1DForOutWhenUnconnected=off
  wires:
  Counter 0 to |b_k|-1/1 -> Subtract/2, Compare To Zero/1, b_k_addr/1
  Subtract/1 -> Data_History_Rd_addr/1
  Input_Addr_Counter/1 -> Rate Transition/1
  Add/1 -> Input_Addr/1
  Constant/1 -> Add/2
  Realignment_delay/1 -> Subtract/3
  Compare To Zero/1 -> End_of_sample_calc/1
  Rate Transition/1 -> Subtract/1, Add/1

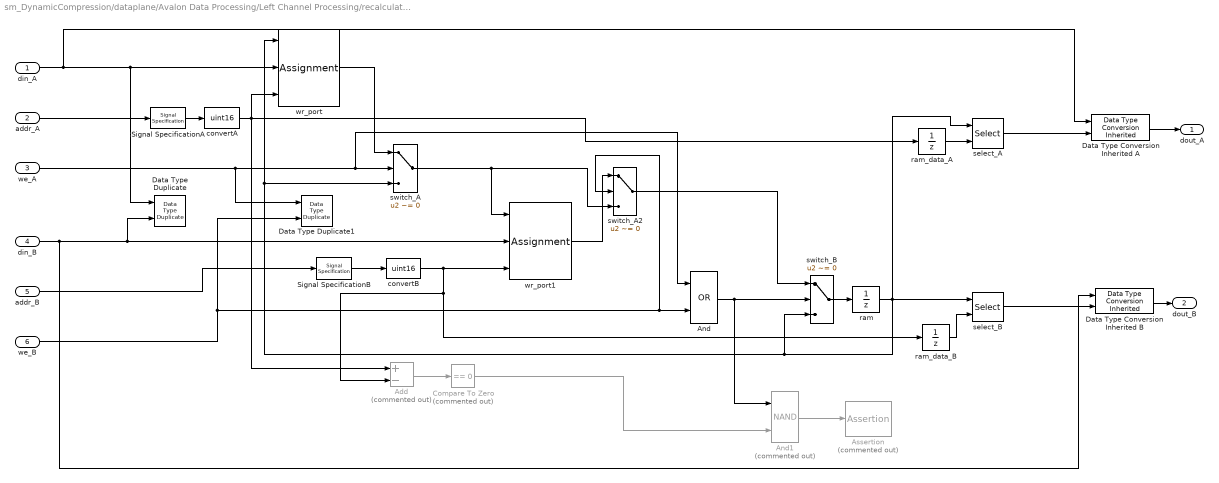
== system sm_DynamicCompression/dataplane/Avalon Data Processing/Left Channel Processing/recalculate/Nchan_FbankAGC_AID/Static_pFIR/B_k_Memory_Block ==
  din_A : Inport
  addr_A : Inport  Port=2
  we_A : Inport  Port=3  OutDataTypeStr=boolean
  din_B : Inport  Port=4
  addr_B : Inport  Port=5
  we_B : Inport  Port=6  OutDataTypeStr=boolean
  Add : Sum  Commented=on  Inputs=+-
  And : Logic  Operator=OR  AllPortsSameDT=off  OutDataTypeStr=boolean
  And1 : Logic  Commented=on  Operator=NAND  AllPortsSameDT=off  OutDataTypeStr=boolean
  Assertion : Assertion  Commented=on  StopWhenAssertionFail=off
  Compare To Zero : simulink/Logic and Bit Operations/Compare To Zero  Commented=on  relop===  OutDataTypeStr=boolean
  Data Type Conversion Inherited A : simulink/Signal Attributes/Data Type Conversion Inherited  ConvertRealWorld=Real World Value  DoSatur=off
      settings: SourceProductName=Simulink  SourceProductBaseCode=SL
  Data Type Conversion Inherited B : simulink/Signal Attributes/Data Type Conversion Inherited  ConvertRealWorld=Real World Value  DoSatur=off
      settings: SourceProductName=Simulink  SourceProductBaseCode=SL
  Data Type Duplicate : DataTypeDuplicate
  Data Type Duplicate1 : DataTypeDuplicate
  Signal SpecificationA : SignalSpecification  OutDataTypeStr=fixdt(0,ram_size,0)  Dimensions=1
  Signal SpecificationB : SignalSpecification  OutDataTypeStr=fixdt(0,ram_size,0)  Dimensions=1
  convertA : DataTypeConversion  OutDataTypeStr=uint16
  convertB : DataTypeConversion  OutDataTypeStr=uint16
  ram : UnitDelay  InitialCondition=B_k_0_init  SampleTime=-1  HasFrameUpgradeWarning=on
  ram_data_A : UnitDelay  SampleTime=-1  HasFrameUpgradeWarning=on
  ram_data_B : UnitDelay  SampleTime=-1  HasFrameUpgradeWarning=on
  select_A : Selector  IndexMode=Zero-based  InputPortWidth=2^ram_size  IndexOptions=Index vector (port)  Indices=[1 3]  OutputSizes=1
  select_B : Selector  IndexMode=Zero-based  InputPortWidth=2^ram_size  IndexOptions=Index vector (port)  Indices=[1 3]  OutputSizes=1
  switch_A : Switch  Criteria=u2 ~= 0
  switch_A2 : Switch  Criteria=u2 ~= 0
  switch_B : Switch  Criteria=u2 ~= 0
  wr_port : Assignment  IndexMode=Zero-based  IndexOptions=Index vector (port)  Indices=1  OutputSizes=[1 1]
  wr_port1 : Assignment  IndexMode=Zero-based  IndexOptions=Index vector (port)  Indices=1  OutputSizes=[1 1]
  dout_A : Outport  VectorParamsAs1DForOutWhenUnconnected=off
  dout_B : Outport  Port=2  VectorParamsAs1DForOutWhenUnconnected=off
  wires:
  switch_A2/1 -> switch_B/1
  And1/1 -> Assertion/1
  Signal SpecificationA/1 -> convertA/1
  Signal SpecificationB/1 -> convertB/1
  switch_B/1 -> ram/1
  convertA/1 -> ram_data_A/1, wr_port/3, Add/1
  ram/1 -> select_B/1, switch_B/3, switch_A/3, wr_port/1, select_A/1
  wr_port/1 -> switch_A/1
  And/1 -> And1/1, switch_B/2
  wr_port1/1 -> switch_A2/1
  Add/1 -> Compare To Zero/1
  Compare To Zero/1 -> And1/2
  we_B/1 -> switch_A2/2, And/2, Data Type Duplicate1/2
  switch_A/1 -> wr_port1/1, switch_A2/3
  addr_B/1 -> Signal SpecificationB/1
  ram_data_B/1 -> select_B/2
  we_A/1 -> Data Type Duplicate1/1, And/1, switch_A/2
  ram_data_A/1 -> select_A/2
  din_A/1 -> Data Type Duplicate/1, wr_port/2, Data Type Conversion Inherited A/1
  convertB/1 -> ram_data_B/1, Add/2, wr_port1/3
  din_B/1 -> wr_port1/2, Data Type Duplicate/2, Data Type Conversion Inherited B/1
  addr_A/1 -> Signal SpecificationA/1
  select_B/1 -> Data Type Conversion Inherited B/2
  Data Type Conversion Inherited B/1 -> dout_B/1
  select_A/1 -> Data Type Conversion Inherited A/2
  Data Type Conversion Inherited A/1 -> dout_A/1
